simulink model "SP_5BandEqualizer"  (Simulink 7.3)
settings: Solver=ode45  StartTime=0.0  StopTime=inf  RelTol=1e-3
values from neighbouring files (symbols this model uses):
  fSampling = 22050    [SP_4BandEqualizer.mat]
undefined symbols (not defined in the file or in its folder): dfilt
libraries: simulink x30, dsparch4 x3, dspsrcs4 x2, dspsnks4 x2
settings Model: Creator=kmodi  LastModifiedBy=kmodi

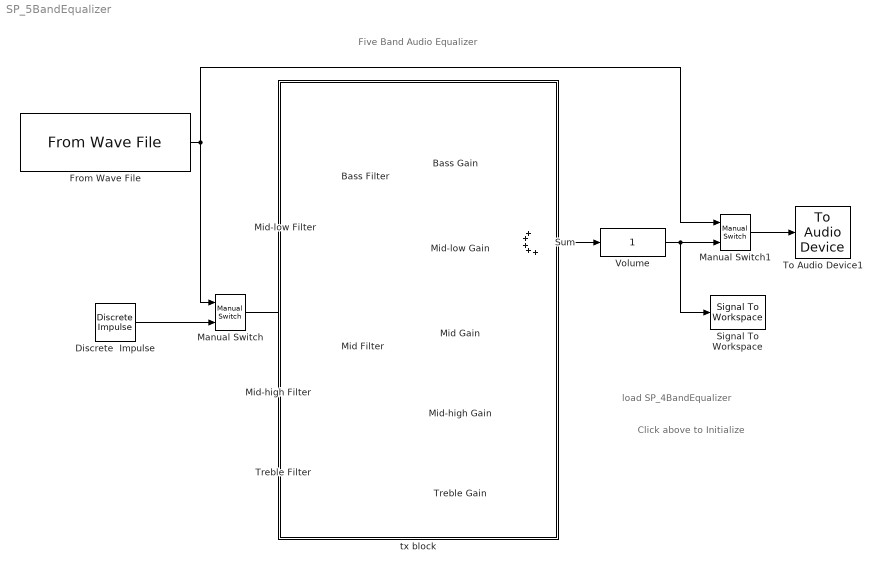
== system SP_5BandEqualizer ==
  note: Five Band Audio Equalizer
  note: load SP_4BandEqualizer
  note: Click above to Initialize
  Bass Filter : dsparch4/Digital Filter  DialogController=dspdialog.DigitalFilter  DialogControllerArgs=DataTag0  TypePopup=IIR (poles & zeros)  IIRFiltStruct=Direct form II transposed  AllPoleFiltStruct=Direct form  FIRFiltStruct=Direct form  CoeffSource=Specify via dialog  NumCoeffs=numLP  DenCoeffs=denLP  BiQuadCoeffs=[1 0.3 0.4 1 0.1 0.2]  LatticeCoeffs=[0.2 0.4]  denIgnore=on  FiltPerSampPopup=One filter per frame  IC=0  ICnum=0  ICden=0  roundingMode=Floor  overflowMode=off  ScaleValues=1  scaleValueFracLength=14  stageInFracLength=15  stageOutFracLength=15  FilterSource=Specify via dialog  dfiltObjectName=dfilt.dffir([1 2 1])
  Bass Gain : simulink/Math Operations/Slider Gain  SystemSampleTime=-1  low=0  gain=1  high=2
  Discrete  Impulse : dspsrcs4/Discrete  Impulse  Delay=0  SampleTime=1/fSampling  FrameSample=1  dataType=double  isSigned=on  wordLen=16  udDataType=sfix(16)  fracBitsMode=Best precision  numFracBits=15
  From Wave File : dspsrcs4/From Wave File  FileName=myRecord  SamplesPerFrame=1  MinBufSize=256  dType=double  bLoop=on  timesToPlay=1000  restartMode=immediately after last sample  firstSampleOutput=off  lastSampleOutput=off
  Manual Switch : simulink/Signal Routing/Manual Switch  SystemSampleTime=-1  sw=1  action=0  varsize=off
  Manual Switch1 : simulink/Signal Routing/Manual Switch  SystemSampleTime=-1  sw=0  action=0  varsize=off
  Mid Filter : dsparch4/Digital Filter  DialogController=dspdialog.DigitalFilter  DialogControllerArgs=DataTag1  TypePopup=IIR (poles & zeros)  IIRFiltStruct=Direct form II transposed  AllPoleFiltStruct=Direct form  FIRFiltStruct=Direct form  CoeffSource=Specify via dialog  NumCoeffs=numMid2  DenCoeffs=denMid2  BiQuadCoeffs=[1 0.3 0.4 1 0.1 0.2]  LatticeCoeffs=[0.2 0.4]  denIgnore=on  FiltPerSampPopup=One filter per frame  IC=0  ICnum=0  ICden=0  roundingMode=Floor  overflowMode=off  ScaleValues=1  scaleValueFracLength=14  stageInFracLength=15  stageOutFracLength=15  FilterSource=Specify via dialog  dfiltObjectName=dfilt.dffir([1 2 1])
  Mid Gain : simulink/Math Operations/Slider Gain  SystemSampleTime=-1  low=0  gain=0  high=2
  Mid-high Filter : dsparch4/Digital Filter  DialogController=dspdialog.DigitalFilter  DialogControllerArgs=DataTag2  TypePopup=FIR (all zeros)  IIRFiltStruct=Direct form II transposed  AllPoleFiltStruct=Direct form  FIRFiltStruct=Direct form  CoeffSource=Specify via dialog  NumCoeffs=numMid3  DenCoeffs=denMid2  BiQuadCoeffs=[1 0.3 0.4 1 0.1 0.2]  LatticeCoeffs=[0.2 0.4]  denIgnore=on  FiltPerSampPopup=One filter per frame  IC=0  ICnum=0  ICden=0  roundingMode=Floor  overflowMode=off  ScaleValues=1  scaleValueFracLength=14  stageInFracLength=15  stageOutFracLength=15  FilterSource=Specify via dialog  dfiltObjectName=dfilt.dffir([1 2 1])
  Mid-high Gain : simulink/Math Operations/Slider Gain  SystemSampleTime=-1  low=0  gain=0  high=2
  Mid-low Filter : Subsystem  Tag=FilterWizardSubSystem
      settings: ErrorFcn=dspFilterRealizedInBasicElemsAlgLoopErrFcnCallback
  Mid-low Gain : simulink/Math Operations/Slider Gain  SystemSampleTime=-1  low=0  gain=0  high=2
  Signal To Workspace : dspsnks4/Signal To Workspace  SystemSampleTime=-1  VariableName=yout  FrameMode=Concatenate frames (2-D array)
      settings: FixptAsFi=off
  Sum : Sum  Inputs=|+++++  OutDataType=fixdt(1, 16)  OutScaling=2^0
  To Audio Device1 : dspsnks4/To Audio Device  DialogController=dspDDGCreate  DialogControllerArgs=DataTag4  deviceName=Default  inheritSampleRate=off  sampleRate=22050  deviceDatatype=Determine from input data type  autoBufferSize=on  bufferSize=4096  queueDuration=1.0
  Treble Filter : Subsystem  Tag=FilterWizardSubSystem
      settings: ErrorFcn=dspFilterRealizedInBasicElemsAlgLoopErrFcnCallback
  Treble Gain : simulink/Math Operations/Slider Gain  SystemSampleTime=-1  low=0  gain=1  high=2
  "Volume " : simulink/Math Operations/Slider Gain  SystemSampleTime=-1  low=0  gain=1  high=2
  tx block : Subsystem
      mask Display: disp('')
  wires:
  Bass Filter/1 -> Bass Gain/1
  Mid-low Filter/1(Output) -> Mid-low Gain/1
  Sum/1 -> "Volume "/1
  Bass Gain/1 -> Sum/1
  Mid-low Gain/1 -> Sum/2
  "Volume "/1 -> Signal To Workspace/1, Manual Switch1/2
  Mid Filter/1 -> Mid Gain/1
  Mid Gain/1 -> Sum/3
  Mid-high Filter/1 -> Mid-high Gain/1
  Mid-high Gain/1 -> Sum/4
  From Wave File/1 -> Manual Switch/1, Manual Switch1/1
  Manual Switch/1 -> Mid Filter/1, Mid-low Filter/1(Input), Bass Filter/1, Mid-high Filter/1, Treble Filter/1(Input)
  Discrete  Impulse/1 -> Manual Switch/2
  Manual Switch1/1 -> To Audio Device1/1
  Treble Filter/1(Output) -> Treble Gain/1
  Treble Gain/1 -> Sum/5

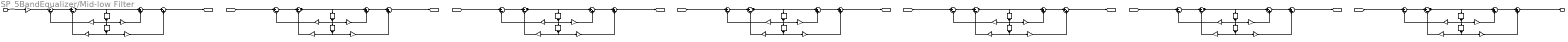
== system SP_5BandEqualizer/Mid-low Filter ==
  Input : Inport
  Delay{11..17,21..27} (14 alike) : simulink/Discrete/Integer Delay  vinit=0.0  samptime=-1  NumDelays=1
  SumA{21..27,31..37} (14 alike) : Sum  Inputs=|+-  OutScaling=1  RndMeth=Nearest  SaturateOnIntegerOverflow=on  OutDataTypeStr=Inherit: Same as first input
  SumB{21..27,31..37} (14 alike) : Sum  Inputs=|++  OutScaling=1  RndMeth=Nearest  SaturateOnIntegerOverflow=on  OutDataTypeStr=Inherit: Same as first input
  a(2)(1) : Gain  Gain=-1.8397589147605165  ParameterDataTypeMode=Specify via dialog  ParameterDataType=float('double')  ParamDataTypeStr=float('double')  OutScaling=1  RndMeth=Nearest  SaturateOnIntegerOverflow=on  OutDataTypeStr=Inherit: Same as input
  a(2)(2) : Gain  Gain=-1.8583220864166883  ParameterDataTypeMode=Specify via dialog  ParameterDataType=float('double')  ParamDataTypeStr=float('double')  OutScaling=1  RndMeth=Nearest  SaturateOnIntegerOverflow=on  OutDataTypeStr=Inherit: Same as input
  a(2)(3) : Gain  Gain=-1.8712688014443435  ParameterDataTypeMode=Specify via dialog  ParameterDataType=float('double')  ParamDataTypeStr=float('double')  OutScaling=1  RndMeth=Nearest  SaturateOnIntegerOverflow=on  OutDataTypeStr=Inherit: Same as input
  a(2)(4) : Gain  Gain=-1.9069399167069183  ParameterDataTypeMode=Specify via dialog  ParameterDataType=float('double')  ParamDataTypeStr=float('double')  OutScaling=1  RndMeth=Nearest  SaturateOnIntegerOverflow=on  OutDataTypeStr=Inherit: Same as input
  a(2)(5) : Gain  Gain=-1.9471940030405648  ParameterDataTypeMode=Specify via dialog  ParameterDataType=float('double')  ParamDataTypeStr=float('double')  OutScaling=1  RndMeth=Nearest  SaturateOnIntegerOverflow=on  OutDataTypeStr=Inherit: Same as input
  a(2)(6) : Gain  Gain=-1.926593286699446  ParameterDataTypeMode=Specify via dialog  ParameterDataType=float('double')  ParamDataTypeStr=float('double')  OutScaling=1  RndMeth=Nearest  SaturateOnIntegerOverflow=on  OutDataTypeStr=Inherit: Same as input
  a(2)(7) : Gain  Gain=-1.9782662654393  ParameterDataTypeMode=Specify via dialog  ParameterDataType=float('double')  ParamDataTypeStr=float('double')  OutScaling=1  RndMeth=Nearest  SaturateOnIntegerOverflow=on  OutDataTypeStr=Inherit: Same as input
  a(3)(1) : Gain  Gain=0.86739367596745631  ParameterDataTypeMode=Specify via dialog  ParameterDataType=float('double')  ParamDataTypeStr=float('double')  OutScaling=1  RndMeth=Nearest  SaturateOnIntegerOverflow=on  OutDataTypeStr=Inherit: Same as input
  a(3)(2) : Gain  Gain=0.87513761574710858  ParameterDataTypeMode=Specify via dialog  ParameterDataType=float('double')  ParamDataTypeStr=float('double')  OutScaling=1  RndMeth=Nearest  SaturateOnIntegerOverflow=on  OutDataTypeStr=Inherit: Same as input
  a(3)(3) : Gain  Gain=0.90766844036617067  ParameterDataTypeMode=Specify via dialog  ParameterDataType=float('double')  ParamDataTypeStr=float('double')  OutScaling=1  RndMeth=Nearest  SaturateOnIntegerOverflow=on  OutDataTypeStr=Inherit: Same as input
  a(3)(4) : Gain  Gain=0.91734710412163789  ParameterDataTypeMode=Specify via dialog  ParameterDataType=float('double')  ParamDataTypeStr=float('double')  OutScaling=1  RndMeth=Nearest  SaturateOnIntegerOverflow=on  OutDataTypeStr=Inherit: Same as input
  a(3)(5) : Gain  Gain=0.95541312807765288  ParameterDataTypeMode=Specify via dialog  ParameterDataType=float('double')  ParamDataTypeStr=float('double')  OutScaling=1  RndMeth=Nearest  SaturateOnIntegerOverflow=on  OutDataTypeStr=Inherit: Same as input
  a(3)(6) : Gain  Gain=0.96761068739952549  ParameterDataTypeMode=Specify via dialog  ParameterDataType=float('double')  ParamDataTypeStr=float('double')  OutScaling=1  RndMeth=Nearest  SaturateOnIntegerOverflow=on  OutDataTypeStr=Inherit: Same as input
  a(3)(7) : Gain  Gain=0.98590111868989483  ParameterDataTypeMode=Specify via dialog  ParameterDataType=float('double')  ParamDataTypeStr=float('double')  OutScaling=1  RndMeth=Nearest  SaturateOnIntegerOverflow=on  OutDataTypeStr=Inherit: Same as input
  b(2)(1) : Gain  Gain=1.318944953254686e-013  ParameterDataTypeMode=Specify via dialog  ParameterDataType=float('double')  ParamDataTypeStr=float('double')  OutScaling=1  RndMeth=Nearest  SaturateOnIntegerOverflow=on  OutDataTypeStr=Inherit: Same as input
  b(2)(2) : Gain  Gain=-1.6432990603581503  ParameterDataTypeMode=Specify via dialog  ParameterDataType=float('double')  ParamDataTypeStr=float('double')  OutScaling=1  RndMeth=Nearest  SaturateOnIntegerOverflow=on  OutDataTypeStr=Inherit: Same as input
  b(2)(3) : Gain  Gain=-1.8614317424464004  ParameterDataTypeMode=Specify via dialog  ParameterDataType=float('double')  ParamDataTypeStr=float('double')  OutScaling=1  RndMeth=Nearest  SaturateOnIntegerOverflow=on  OutDataTypeStr=Inherit: Same as input
  b(2)(4) : Gain  Gain=-1.9991713736623455  ParameterDataTypeMode=Specify via dialog  ParameterDataType=float('double')  ParamDataTypeStr=float('double')  OutScaling=1  RndMeth=Nearest  SaturateOnIntegerOverflow=on  OutDataTypeStr=Inherit: Same as input
  b(2)(5) : Gain  Gain=-1.9977400579240996  ParameterDataTypeMode=Specify via dialog  ParameterDataType=float('double')  ParamDataTypeStr=float('double')  OutScaling=1  RndMeth=Nearest  SaturateOnIntegerOverflow=on  OutDataTypeStr=Inherit: Same as input
  b(2)(6) : Gain  Gain=-1.8991207395228842  ParameterDataTypeMode=Specify via dialog  ParameterDataType=float('double')  ParamDataTypeStr=float('double')  OutScaling=1  RndMeth=Nearest  SaturateOnIntegerOverflow=on  OutDataTypeStr=Inherit: Same as input
  b(2)(7) : Gain  Gain=-1.9968661186880208  ParameterDataTypeMode=Specify via dialog  ParameterDataType=float('double')  ParamDataTypeStr=float('double')  OutScaling=1  RndMeth=Nearest  SaturateOnIntegerOverflow=on  OutDataTypeStr=Inherit: Same as input
  b(3)(1) : Gain  Gain=-1.0000000000001319  ParameterDataTypeMode=Specify via dialog  ParameterDataType=float('double')  ParamDataTypeStr=float('double')  OutScaling=1  RndMeth=Nearest  SaturateOnIntegerOverflow=on  OutDataTypeStr=Inherit: Same as input
  b(3)(2) : Gain  Gain=1.0000000000000222  ParameterDataTypeMode=Specify via dialog  ParameterDataType=float('double')  ParamDataTypeStr=float('double')  OutScaling=1  RndMeth=Nearest  SaturateOnIntegerOverflow=on  OutDataTypeStr=Inherit: Same as input
  b(3)(3) : Gain  Gain=1.0000000000000007  ParameterDataTypeMode=Specify via dialog  ParameterDataType=float('double')  ParamDataTypeStr=float('double')  OutScaling=1  RndMeth=Nearest  SaturateOnIntegerOverflow=on  OutDataTypeStr=Inherit: Same as input
  b(3)(4) : Gain  Gain=1.000000000000002  ParameterDataTypeMode=Specify via dialog  ParameterDataType=float('double')  ParamDataTypeStr=float('double')  OutScaling=1  RndMeth=Nearest  SaturateOnIntegerOverflow=on  OutDataTypeStr=Inherit: Same as input
  b(3)(5) : Gain  Gain=1.0000000000000024  ParameterDataTypeMode=Specify via dialog  ParameterDataType=float('double')  ParamDataTypeStr=float('double')  OutScaling=1  RndMeth=Nearest  SaturateOnIntegerOverflow=on  OutDataTypeStr=Inherit: Same as input
  b(3)(6) : Gain  Gain=1.0000000000000002  ParameterDataTypeMode=Specify via dialog  ParameterDataType=float('double')  ParamDataTypeStr=float('double')  OutScaling=1  RndMeth=Nearest  SaturateOnIntegerOverflow=on  OutDataTypeStr=Inherit: Same as input
  b(3)(7) : Gain  Gain=0.99999999999999989  ParameterDataTypeMode=Specify via dialog  ParameterDataType=float('double')  ParamDataTypeStr=float('double')  OutScaling=1  RndMeth=Nearest  SaturateOnIntegerOverflow=on  OutDataTypeStr=Inherit: Same as input
  s(1) : Gain  Gain=7.7919570257835674e-005  ParameterDataTypeMode=Specify via dialog  ParameterDataType=float('double')  ParamDataTypeStr=float('double')  OutScaling=1  RndMeth=Nearest  SaturateOnIntegerOverflow=on  OutDataTypeStr=Inherit: Same as input
  Output : Outport
  wires:
  b(3)(7)/1 -> SumB37/2
  Delay27/1 -> b(3)(7)/1, a(3)(7)/1
  a(3)(7)/1 -> SumA37/2
  b(2)(7)/1 -> SumB27/2
  Delay17/1 -> Delay27/1, b(2)(7)/1, a(2)(7)/1
  a(2)(7)/1 -> SumA27/2
  SumB37/1 -> Output/1
  SumB27/1 -> SumB37/1
  SumA37/1 -> Delay17/1, SumB27/1
  SumA27/1 -> SumA37/1
  [Sect6] -> SumA27/1
  b(3)(6)/1 -> SumB36/2
  Delay26/1 -> b(3)(6)/1, a(3)(6)/1
  a(3)(6)/1 -> SumA36/2
  b(2)(6)/1 -> SumB26/2
  Delay16/1 -> Delay26/1, b(2)(6)/1, a(2)(6)/1
  a(2)(6)/1 -> SumA26/2
  SumB36/1 -> [Sect6]
  SumB26/1 -> SumB36/1
  SumA36/1 -> Delay16/1, SumB26/1
  SumA26/1 -> SumA36/1
  [Sect5] -> SumA26/1
  b(3)(5)/1 -> SumB35/2
  Delay25/1 -> b(3)(5)/1, a(3)(5)/1
  a(3)(5)/1 -> SumA35/2
  b(2)(5)/1 -> SumB25/2
  Delay15/1 -> Delay25/1, b(2)(5)/1, a(2)(5)/1
  a(2)(5)/1 -> SumA25/2
  SumB35/1 -> [Sect5]
  SumB25/1 -> SumB35/1
  SumA35/1 -> Delay15/1, SumB25/1
  SumA25/1 -> SumA35/1
  [Sect4] -> SumA25/1
  b(3)(4)/1 -> SumB34/2
  Delay24/1 -> b(3)(4)/1, a(3)(4)/1
  a(3)(4)/1 -> SumA34/2
  b(2)(4)/1 -> SumB24/2
  Delay14/1 -> Delay24/1, b(2)(4)/1, a(2)(4)/1
  a(2)(4)/1 -> SumA24/2
  SumB34/1 -> [Sect4]
  SumB24/1 -> SumB34/1
  SumA34/1 -> Delay14/1, SumB24/1
  SumA24/1 -> SumA34/1
  [Sect3] -> SumA24/1
  b(3)(3)/1 -> SumB33/2
  Delay23/1 -> b(3)(3)/1, a(3)(3)/1
  a(3)(3)/1 -> SumA33/2
  b(2)(3)/1 -> SumB23/2
  Delay13/1 -> Delay23/1, b(2)(3)/1, a(2)(3)/1
  a(2)(3)/1 -> SumA23/2
  SumB33/1 -> [Sect3]
  SumB23/1 -> SumB33/1
  SumA33/1 -> Delay13/1, SumB23/1
  SumA23/1 -> SumA33/1
  [Sect2] -> SumA23/1
  b(3)(2)/1 -> SumB32/2
  Delay22/1 -> b(3)(2)/1, a(3)(2)/1
  a(3)(2)/1 -> SumA32/2
  b(2)(2)/1 -> SumB22/2
  Delay12/1 -> Delay22/1, b(2)(2)/1, a(2)(2)/1
  a(2)(2)/1 -> SumA22/2
  SumB32/1 -> [Sect2]
  SumB22/1 -> SumB32/1
  SumA32/1 -> Delay12/1, SumB22/1
  SumA22/1 -> SumA32/1
  [Sect1] -> SumA22/1
  b(3)(1)/1 -> SumB31/2
  Delay21/1 -> b(3)(1)/1, a(3)(1)/1
  a(3)(1)/1 -> SumA31/2
  b(2)(1)/1 -> SumB21/2
  Delay11/1 -> Delay21/1, b(2)(1)/1, a(2)(1)/1
  a(2)(1)/1 -> SumA21/2
  SumB31/1 -> [Sect1]
  SumB21/1 -> SumB31/1
  SumA31/1 -> Delay11/1, SumB21/1
  SumA21/1 -> SumA31/1
  s(1)/1 -> SumA21/1
  Input/1 -> s(1)/1

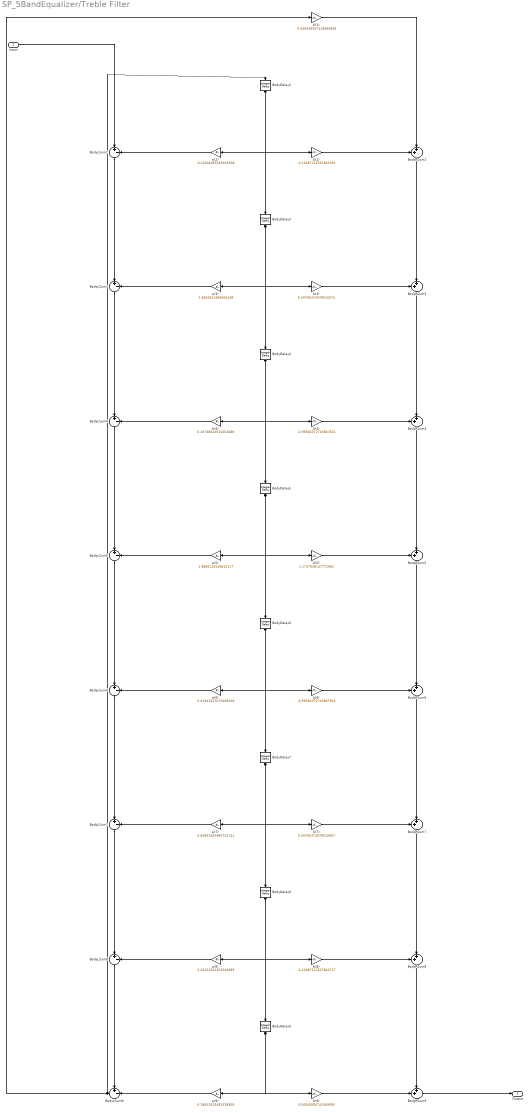
== system SP_5BandEqualizer/Treble Filter ==
  Input : Inport
  BodyDelay{2..9} (8 alike) : simulink/Discrete/Integer Delay  vinit=0.0  samptime=-1  NumDelays=1
  BodyLSum{2..8} (7 alike) : Sum  Inputs=|+-  OutScaling=1  RndMeth=Nearest  SaturateOnIntegerOverflow=on  OutDataTypeStr=Inherit: Same as first input
  BodyLSum9 : Sum  Inputs=+-|  OutScaling=1  RndMeth=Nearest  SaturateOnIntegerOverflow=on  OutDataTypeStr=Inherit: Same as first input
  BodyRSum{2..9} (8 alike) : Sum  Inputs=++|  OutScaling=1  RndMeth=Nearest  SaturateOnIntegerOverflow=on  OutDataTypeStr=Inherit: Same as first input
  a(2) : Gain  Gain=-0.23004065549035696  ParameterDataTypeMode=Specify via dialog  ParameterDataType=float('double')  ParamDataTypeStr=float('double')  OutScaling=1  RndMeth=Nearest  SaturateOnIntegerOverflow=on  OutDataTypeStr=Inherit: Same as input
  a(3) : Gain  Gain=2.3604621460660438  ParameterDataTypeMode=Specify via dialog  ParameterDataType=float('double')  ParamDataTypeStr=float('double')  OutScaling=1  RndMeth=Nearest  SaturateOnIntegerOverflow=on  OutDataTypeStr=Inherit: Same as input
  a(4) : Gain  Gain=0.20738024531054688  ParameterDataTypeMode=Specify via dialog  ParameterDataType=float('double')  ParamDataTypeStr=float('double')  OutScaling=1  RndMeth=Nearest  SaturateOnIntegerOverflow=on  OutDataTypeStr=Inherit: Same as input
  a(5) : Gain  Gain=1.9866115549810117  ParameterDataTypeMode=Specify via dialog  ParameterDataType=float('double')  ParamDataTypeStr=float('double')  OutScaling=1  RndMeth=Nearest  SaturateOnIntegerOverflow=on  OutDataTypeStr=Inherit: Same as input
  a(6) : Gain  Gain=0.61941637075608258  ParameterDataTypeMode=Specify via dialog  ParameterDataType=float('double')  ParamDataTypeStr=float('double')  OutScaling=1  RndMeth=Nearest  SaturateOnIntegerOverflow=on  OutDataTypeStr=Inherit: Same as input
  a(7) : Gain  Gain=0.84693265986725741  ParameterDataTypeMode=Specify via dialog  ParameterDataType=float('double')  ParamDataTypeStr=float('double')  OutScaling=1  RndMeth=Nearest  SaturateOnIntegerOverflow=on  OutDataTypeStr=Inherit: Same as input
  a(8) : Gain  Gain=0.25221562353240889  ParameterDataTypeMode=Specify via dialog  ParameterDataType=float('double')  ParamDataTypeStr=float('double')  OutScaling=1  RndMeth=Nearest  SaturateOnIntegerOverflow=on  OutDataTypeStr=Inherit: Same as input
  a(9) : Gain  Gain=0.18652620481538909  ParameterDataTypeMode=Specify via dialog  ParameterDataType=float('double')  ParamDataTypeStr=float('double')  OutScaling=1  RndMeth=Nearest  SaturateOnIntegerOverflow=on  OutDataTypeStr=Inherit: Same as input
  b(1) : Gain  Gain=0.049458947416689658  ParameterDataTypeMode=Specify via dialog  ParameterDataType=float('double')  ParamDataTypeStr=float('double')  OutScaling=1  RndMeth=Nearest  SaturateOnIntegerOverflow=on  OutDataTypeStr=Inherit: Same as input
  b(2) : Gain  Gain=-0.23487112507843391  ParameterDataTypeMode=Specify via dialog  ParameterDataType=float('double')  ParamDataTypeStr=float('double')  OutScaling=1  RndMeth=Nearest  SaturateOnIntegerOverflow=on  OutDataTypeStr=Inherit: Same as input
  b(3) : Gain  Gain=0.59795374978510274  ParameterDataTypeMode=Specify via dialog  ParameterDataType=float('double')  ParamDataTypeStr=float('double')  OutScaling=1  RndMeth=Nearest  SaturateOnIntegerOverflow=on  OutDataTypeStr=Inherit: Same as input
  b(4) : Gain  Gain=-0.99582372743807501  ParameterDataTypeMode=Specify via dialog  ParameterDataType=float('double')  ParamDataTypeStr=float('double')  OutScaling=1  RndMeth=Nearest  SaturateOnIntegerOverflow=on  OutDataTypeStr=Inherit: Same as input
  b(5) : Gain  Gain=1.1737938147771962  ParameterDataTypeMode=Specify via dialog  ParameterDataType=float('double')  ParamDataTypeStr=float('double')  OutScaling=1  RndMeth=Nearest  SaturateOnIntegerOverflow=on  OutDataTypeStr=Inherit: Same as input
  b(6) : Gain  Gain=-0.99582372743807945  ParameterDataTypeMode=Specify via dialog  ParameterDataType=float('double')  ParamDataTypeStr=float('double')  OutScaling=1  RndMeth=Nearest  SaturateOnIntegerOverflow=on  OutDataTypeStr=Inherit: Same as input
  b(7) : Gain  Gain=0.59795374978510807  ParameterDataTypeMode=Specify via dialog  ParameterDataType=float('double')  ParamDataTypeStr=float('double')  OutScaling=1  RndMeth=Nearest  SaturateOnIntegerOverflow=on  OutDataTypeStr=Inherit: Same as input
  b(8) : Gain  Gain=-0.23487112507843727  ParameterDataTypeMode=Specify via dialog  ParameterDataType=float('double')  ParamDataTypeStr=float('double')  OutScaling=1  RndMeth=Nearest  SaturateOnIntegerOverflow=on  OutDataTypeStr=Inherit: Same as input
  b(9) : Gain  Gain=0.04945894741669065  ParameterDataTypeMode=Specify via dialog  ParameterDataType=float('double')  ParamDataTypeStr=float('double')  OutScaling=1  RndMeth=Nearest  SaturateOnIntegerOverflow=on  OutDataTypeStr=Inherit: Same as input
  Output : Outport
  wires:
  b(1)/1 -> BodyRSum2/2
  Input/1 -> BodyLSum2/1
  BodyLSum2/1 -> BodyLSum3/1
  a(2)/1 -> BodyLSum2/2
  BodyDelay2/1 -> a(2)/1, b(2)/1, BodyDelay3/1
  b(2)/1 -> BodyRSum2/1
  BodyRSum2/1 -> BodyRSum3/2
  BodyLSum3/1 -> BodyLSum4/1
  a(3)/1 -> BodyLSum3/2
  BodyDelay3/1 -> a(3)/1, b(3)/1, BodyDelay4/1
  b(3)/1 -> BodyRSum3/1
  BodyRSum3/1 -> BodyRSum4/2
  BodyLSum4/1 -> BodyLSum5/1
  a(4)/1 -> BodyLSum4/2
  BodyDelay4/1 -> a(4)/1, b(4)/1, BodyDelay5/1
  b(4)/1 -> BodyRSum4/1
  BodyRSum4/1 -> BodyRSum5/2
  BodyLSum5/1 -> BodyLSum6/1
  a(5)/1 -> BodyLSum5/2
  BodyDelay5/1 -> a(5)/1, b(5)/1, BodyDelay6/1
  b(5)/1 -> BodyRSum5/1
  BodyRSum5/1 -> BodyRSum6/2
  BodyLSum6/1 -> BodyLSum7/1
  a(6)/1 -> BodyLSum6/2
  BodyDelay6/1 -> a(6)/1, b(6)/1, BodyDelay7/1
  b(6)/1 -> BodyRSum6/1
  BodyRSum6/1 -> BodyRSum7/2
  BodyLSum7/1 -> BodyLSum8/1
  a(7)/1 -> BodyLSum7/2
  BodyDelay7/1 -> a(7)/1, b(7)/1, BodyDelay8/1
  b(7)/1 -> BodyRSum7/1
  BodyRSum7/1 -> BodyRSum8/2
  BodyLSum8/1 -> BodyLSum9/1
  a(8)/1 -> BodyLSum8/2
  BodyDelay8/1 -> a(8)/1, b(8)/1, BodyDelay9/1
  b(8)/1 -> BodyRSum8/1
  BodyRSum8/1 -> BodyRSum9/1
  BodyLSum9/1 -> b(1)/1, BodyDelay2/1
  a(9)/1 -> BodyLSum9/2
  BodyDelay9/1 -> a(9)/1, b(9)/1
  b(9)/1 -> BodyRSum9/2
  BodyRSum9/1 -> Output/1

== system SP_5BandEqualizer/tx block ==
